simulink model "blockdemo"  (Simulink 7.0)
settings: Solver=VariableStepDiscrete  StartTime=0  StopTime=300  MaxStep=1  RelTol=1e-3
InitFcn:
  | %% DSPBuilder Start
  | alt_dspbuilder_update_model(bdroot)
  | %% DSPBuilder End
libraries: allblocks_alteradspbuilder2 x5
settings Model: Creator=mjervis  LastModifiedBy=delphick
settings OptimizationCC: BlockReduction=off  BooleanDataType=off  InlineInvariantSignals=on
settings DebuggingCC: SaveWithParameterizedLinksMsg=none  SignalResolutionControl=TryResolveAllWithWarning  SolverPrmCheckMsg=none  MultiTaskDSMMsg=warning  MultiTaskCondExecSysMsg=none
settings HardwareCC: TargetUnknown=on
settings RTWCC: IncludeERTFirstTime=on
settings GRTTargetCC: TargetFcnLib=ansi_tfl_tmw.mat

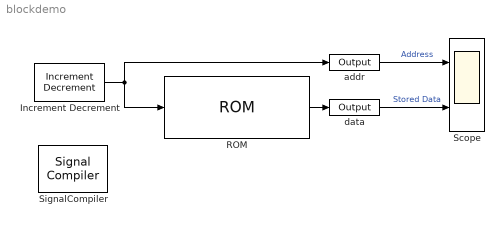
== system blockdemo ==
  Increment Decrement : allblocks_alteradspbuilder2/Increment Decrement  BusType=Signed Integer  bwl=8  bwr=0  SpecifyClock=off  clr_value=0  direction=Increment  phase_selection=1  use_ena=off  use_sclr=off  pipeline_display=1
  ROM : allblocks_alteradspbuilder2/ROM  numwords=2^8  BusType=Signed Fractional  bwl=2  bwr=6  memory_type=AUTO  ram_type=ROM  initialization=From MATLAB array  init_file=unused.hex  init_array=[sin((1/64)*pi*(0:1:255))]  register_outputs=off  use_ena=off  ClockPhase=1  pipeline_display=1  allowFloatingPointOverride=on  logOutputs=off  logFile=C:\perforce_workspace81\main\dsp_builder2\Documentation\DesignExamples\Tutorials\UnitBlocks\Storage\ROM\tb_blockdemo\blockdemo_ROM.fixedpointlog
  Scope : Scope  NumInputPorts=2
      settings: TimeRange=300  YMin=0~-1  YMax=300~1  SampleInput=on  SampleTime=1
  SignalCompiler : allblocks_alteradspbuilder2/Signal Compiler  DeviceFamily=Stratix IV  DeviceName=AUTO  EnableSignalTap=off  SignalTapDepth=128  UseBoardBlock=off  StpUseDefaultClock=on  StpClock=Clock  ExportDir=C:\Documents and Settings\delphick\My Documents\MATLAB
  addr : allblocks_alteradspbuilder2/Output  iofile=C:\perforce_workspace81\main\dsp_builder2\Documentation\DesignExamples\Tutorials\UnitBlocks\Storage\ROM\tb_blockdemo\blockdemo_addr.capture  BusType=Unsigned Integer  bwl=8  bwr=0  externalType=Inferred  PORTTYPE=Output  allowFloatingPointOverride=on  logOutputs=off
  data : allblocks_alteradspbuilder2/Output  iofile=C:\perforce_workspace81\main\dsp_builder2\Documentation\DesignExamples\Tutorials\UnitBlocks\Storage\ROM\tb_blockdemo\blockdemo_data.capture  BusType=Inferred  bwl=8  bwr=0  externalType=Inferred  PORTTYPE=Output  allowFloatingPointOverride=on  logOutputs=off
  wires:
  Increment Decrement/1 -> ROM/1, addr/1
  ROM/1 -> data/1
  addr/1 -> Scope/1  "Address"
  data/1 -> Scope/2  "Stored Data"
